simulink model "EMGRecorder"  (R2019a)
settings: Solver=FixedStepAuto  StartTime=0.0  StopTime=inf  RelTol=1e-3  EnableMultiTasking=on
undefined symbols (not defined in the file or in its folder): daq
libraries: daqlib x2
settings Model: ExtModeTrigDuration=2  Creator=Kusunoki  LastModifiedBy=Owner
settings OptimizationCC: EnhancedBackFolding=on  PassReuseOutputArgsAs=Individual arguments  MaxStackSize=64  OptimizeBlockOrder=speed  DifferentSizesBufferReuse=on  OptimizationCustomize=off
settings DebuggingCC: ParameterTunabilityLossMsg=error
settings HardwareCC: ProdBitPerInt=16  ProdBitPerPointer=16  ProdBitPerSizeT=16  ProdBitPerPtrDiffT=16  ProdLargestAtomicFloat=None  ProdWordSize=8  ProdHWDeviceType=Atmel->AVR
settings SFSimCC: MATLABDynamicMemAlloc=off
settings RTWCC: SystemTargetFile=ert.tlc  HardwareBoard=Arduino Mega 2560  TLCOptions=-aInlineSetEventsForThisBaseRateFcn=TLC_FALSE -aSuppressMultiTaskScheduler=TLC_FALSE -aRateBasedStepFcn=1  TemplateMakefile=ert_default_tmf  GenerateReport=on  Toolchain=Arduino AVR  BuildConfiguration=Faster Runs  IncludeHyperlinkInReport=on  LaunchReport=on  GenerateTraceInfo=on  GenerateTraceReport=on  GenerateTraceReportSl=on  GenerateTraceReportSf=on  GenerateTraceReportEml=on
settings CodeAppCC: ForceParamTrailComments=on  IgnoreCustomStorageClasses=off  OperatorAnnotations=on  SimulinkDataObjDesc=on  SFDataObjDesc=on  InsertBlockDesc=on
settings ERTTargetCC: SupportContinuousTime=on  SupportVariableSizeSignals=on  ExtModeStaticAllocSize=2048

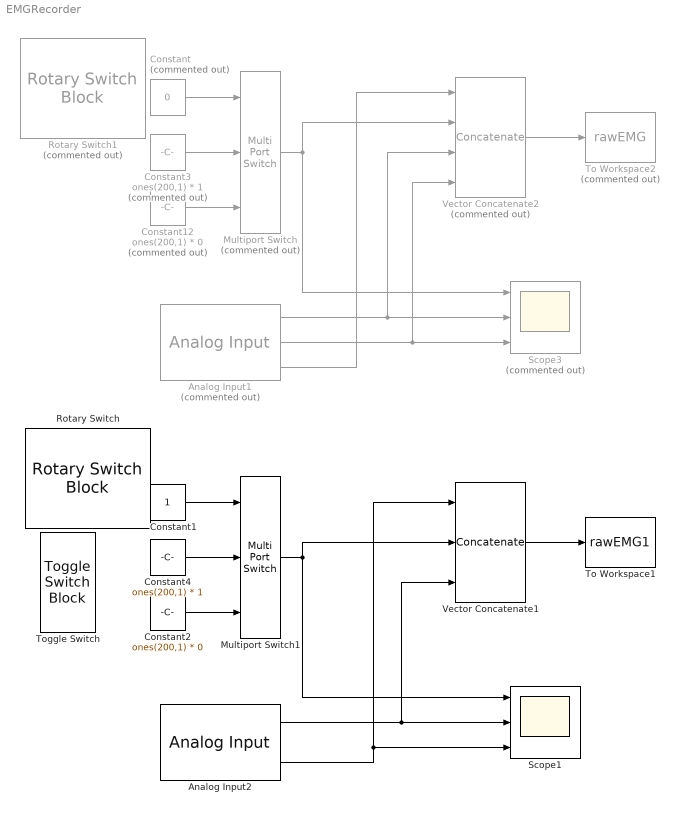
== system EMGRecorder ==
  Analog Input1 : daqlib/Analog Input  Commented=on  DeviceMenu=ni Dev1 (USB-6000)  Device=ni Dev1 (USB-6000)  ObjConstructor=daq.createSession('ni')  NChannelsSelected=2  Channels=1$ai0$$Dev1$1$1$1$1$#1$ai1$$Dev1$1$1$1$1$#0$ai2$$Dev1$1$1$1$1$#0$ai3$$Dev1$1$1$1$1$#0$ai4$$Dev1$1$1$1$1$#0$ai5$$Dev1$1$1$1$1$#0$ai6$$Dev1$1$1$1$1$#0$ai7$$Dev1$1$1$1$1$#  NPorts=1 per channel  SampleRate=2000  ActualRate=2000  ScansPerTrigger=200  OutputTimestamp=on  AcqMode=0  NumFrameBuffer=100  OutputTriggertime=off
      settings: SourceProductName=Data Acquisition Toolbox  SourceProductBaseCode=DA
  Analog Input2 : daqlib/Analog Input  DeviceMenu=ni Dev1 (USB-6000)  Device=ni Dev1 (USB-6000)  ObjConstructor=daq.createSession('ni')  NChannelsSelected=1  Channels=1$ai0$$Dev1$1$1$1$1$#0$ai1$$Dev1$1$1$1$1$#0$ai2$$Dev1$1$1$1$1$#0$ai3$$Dev1$1$1$1$1$#0$ai4$$Dev1$1$1$1$1$#0$ai5$$Dev1$1$1$1$1$#0$ai6$$Dev1$1$1$1$1$#0$ai7$$Dev1$1$1$1$1$#  NPorts=1 per channel  SampleRate=2000  ActualRate=2000  ScansPerTrigger=200  OutputTimestamp=on  AcqMode=0  NumFrameBuffer=100  OutputTriggertime=off
      settings: SourceProductName=Data Acquisition Toolbox  SourceProductBaseCode=DA
  Constant : Constant  Commented=on  Value=0
  Constant1 : Constant
  Constant12 : Constant  Commented=on  Value=ones(200,1) * 0
  Constant2 : Constant  Value=ones(200,1) * 0
  Constant3 : Constant  Commented=on  Value=ones(200,1) * 1
  Constant4 : Constant  Value=ones(200,1) * 1
  Multiport Switch : MultiPortSwitch  Commented=on  DataPortOrder=Specify indices  DataPortIndices={1,0}
  Multiport Switch1 : MultiPortSwitch  DataPortOrder=Specify indices  DataPortIndices={1,0}
  Rotary Switch : RotarySwitchBlock
      settings: Values={{'0：relax', '1 : grip'}, [0 1]}
  Rotary Switch1 : RotarySwitchBlock  Commented=on
      settings: Values={{'0 : relax', '1 : grip'}, [0 1]}
  Scope1 : Scope  NumInputPorts=3
  Scope3 : Scope  Commented=on  NumInputPorts=3
  To Workspace1 : ToWorkspace  VariableName=rawEMG1  SampleTime=-1
      settings: Save2DSignal=2-D array (concatenate along first dimension)
  To Workspace2 : ToWorkspace  Commented=on  VariableName=rawEMG  SampleTime=-1
      settings: Save2DSignal=2-D array (concatenate along first dimension)
  Toggle Switch : ToggleSwitchBlock
      settings: Values={{'0', '1'}, [0 1]}
  Vector Concatenate1 : Concatenate  NumInputs=3  Mode=Multidimensional array  ConcatenateDimension=2
  Vector Concatenate2 : Concatenate  Commented=on  NumInputs=4  Mode=Multidimensional array  ConcatenateDimension=2
  wires:
  Constant12/1 -> Multiport Switch/3
  Multiport Switch/1 -> Vector Concatenate2/2, Scope3/1
  Constant3/1 -> Multiport Switch/2
  Constant/1 -> Multiport Switch/1
  Analog Input1/1 -> Scope3/2, Vector Concatenate2/3
  Analog Input1/2 -> Vector Concatenate2/4, Scope3/3
  Vector Concatenate2/1 -> To Workspace2/1
  Analog Input1/3 -> Vector Concatenate2/1
  Vector Concatenate1/1 -> To Workspace1/1
  Analog Input2/2 -> Vector Concatenate1/1, Scope1/3
  Analog Input2/1 -> Vector Concatenate1/3, Scope1/2
  Multiport Switch1/1 -> Scope1/1, Vector Concatenate1/2
  Constant4/1 -> Multiport Switch1/2
  Constant1/1 -> Multiport Switch1/1
  Constant2/1 -> Multiport Switch1/3
